simulink model "Integrated_noAmb"  (R2023b)
settings: Solver=FixedStepAuto  StartTime=0.0  StopTime=16500  FixedStep=2  RelTol=1e-3
settings Model: PacingRate=1000  Creator=20181234  LastModifiedBy=20181234
settings ModelReferenceCC: ModelReferenceMinAlgLoopOccurrences=on

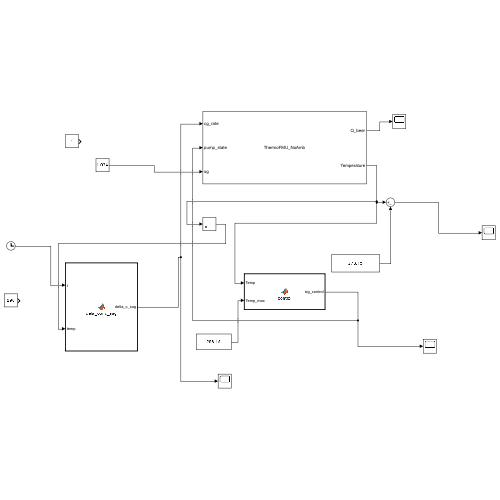
[thumbnail: Simulink's stored preview of the top-level diagram]
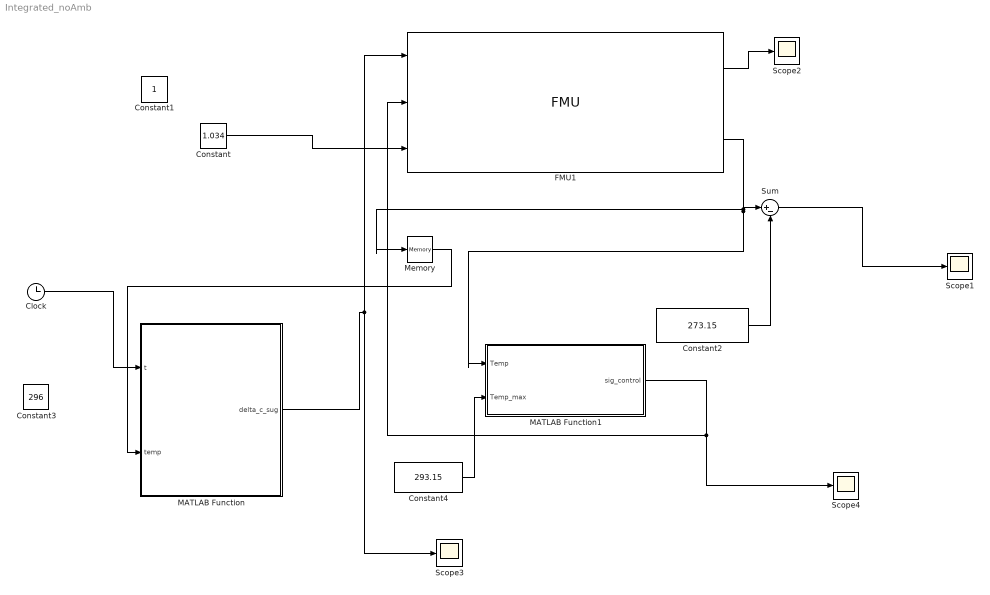
== system Integrated_noAmb ==
  Clock : Clock
  Constant : Constant  Value=1.034
  Constant1 : Constant
  Constant2 : Constant  Value=273.15
  Constant3 : Constant  Value=296
  Constant4 : Constant  Value=293.15
  FMU1 : FMU  FMUName=ThermoFMU_NoAmb.fmu  FMUMode=ModelExchange  FMUIsToleranceUsed=on  FMUToleranceValue=1  FMUInitializeEnumObject=off  FMUCachedDialogLayout="{\"Geometry\":[977,129,436,461],\"ParameterColumnsWidthConfig\":\"{\\\"columns\\\":[{\\\"name\\\":\\\"Parameter\\\",\\\"width\\\":119},{\\\"name\\\":\\\"Value\\\",\\\"width\\\":90},{\\\"name\\\":\\\"Unit\\\",\\\"width\\\":82},{\\\"name\\\":\\\"Description\\\",\\\"width\\\":125}]}\",\"InputColumnsWidthConfig\":[],\"OutputColumnsWidthConfig\":[]}"  A_coil=0.1817  Cp=1.2552  T_0=291.15  T_pump=291.15  Volume=25.0  dH=91200.0  h=200.89  mask(ThermoFMU_NoAmb [Model Exchange, v2.0]){}
      settings: MultithreadedSim=off
      mask Display:
      | disp('ThermoFMU_NoAmb');
      | port_label('output',1,'Q_beer');
      | port_label('output',2,'Temperature');
      | port_label('input',1,'cg_rate');
      | port_label('input',2,'pump_state');
      | port_label('input',3,'sg');
  MATLAB Function : MATLAB Function  TreatAsAtomicUnit=on
  MATLAB Function1 : MATLAB Function  TreatAsAtomicUnit=on
  Memory : Memory  InitialCondition=291.15
  Scope{1..4} (4 alike) : Scope
  Sum : Sum  Inputs=|+-
  wires:
  MATLAB Function1/1(sig_control) -> FMU1/2, Scope4/1
  Constant2/1 -> Sum/2
  Sum/1 -> Scope1/1
  Clock/1 -> MATLAB Function/1(t)
  MATLAB Function/1(delta_c_sug) -> FMU1/1, Scope3/1
  Constant4/1 -> MATLAB Function1/2(Temp_max)
  Constant/1 -> FMU1/3
  FMU1/2 -> Memory/1, MATLAB Function1/1(Temp), Sum/1
  FMU1/1 -> Scope2/1
  Memory/1 -> MATLAB Function/2(temp)

== matlab function Integrated_noAmb/MATLAB Function ==
  data: t input; delta_c_sug output; temp input
function delta_c_sug = dela_conc_sug(t,temp)
A = 1.24503386e-22;
E = -9.35902242e4;
m = -0.000132816;
b = -0.058764065;
R = 8.314; %j/molK

c1=A*exp(-E/(R*temp));
c2=m*temp + b;

delta_c_sug = 2*c1*t+c2;
if delta_c_sug >= 0
    delta_c_sug = 0;
end

== matlab function Integrated_noAmb/MATLAB Function1 ==
  data: Temp input; sig_control output; Temp_max input
function sig_control = control(Temp, Temp_max)


if Temp > Temp_max
    sig_control = 1;
else
    sig_control =0;

end
